simulink model "Empty_Model"  (R2024b)
settings: Solver=FixedStepDiscrete  StartTime=0.0  StopTime=inf  FixedStep=0.01  RelTol=1e-3
libraries: simulink x3, Lib_Model x3
settings Model: PacingRate=0.250000  Creator=HHI  LastModifiedBy=HHI

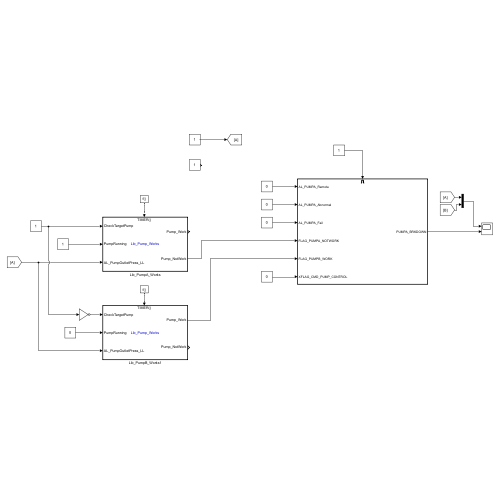
[thumbnail: Simulink's stored preview of the top-level diagram]
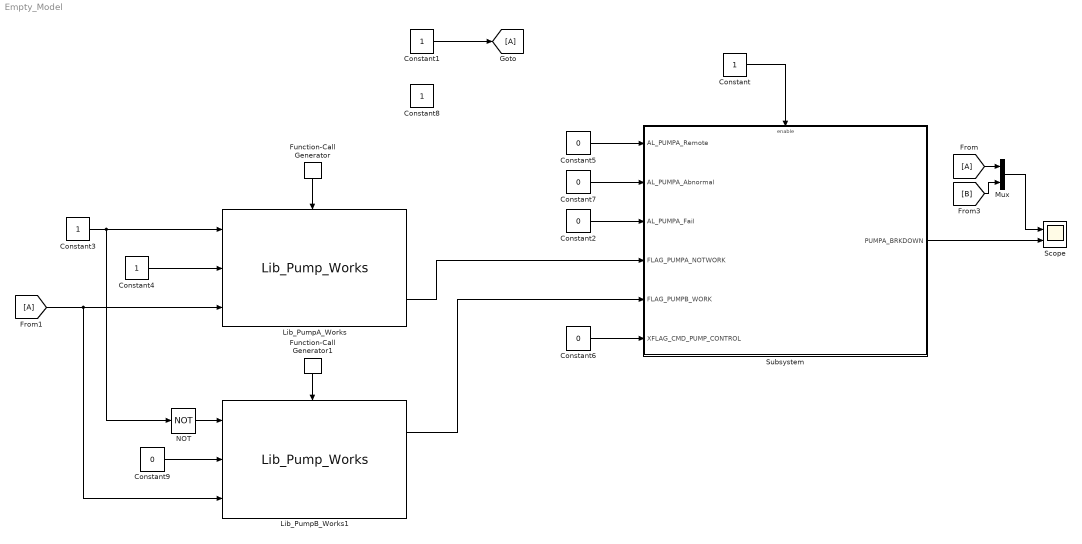
== system Empty_Model ==
  Constant{,1,3..4,8} (5 alike) : Constant  OutDataTypeStr=boolean
  Constant{2,5..7,9} (5 alike) : Constant  Value=0  OutDataTypeStr=boolean
  From : From
  From1 : From
  Function-Call Generator : simulink/Ports & Subsystems/Function-Call Generator  sample_time=1  numberOfIterations=1  DisallowWideOutput=off
  Function-Call Generator1 : simulink/Ports & Subsystems/Function-Call Generator  sample_time=1  numberOfIterations=1  DisallowWideOutput=off
  Goto : Goto
  Lib_PumpA_Works : Lib_Model/Lib_Pump_Works  SystemSampleTime=-1  VariantActivationTime=update diagram  AllowFlexibleInterface=on  Latency=0  AutoFrameSizeCalculation=off
  Lib_PumpB_Works1 : Lib_Model/Lib_Pump_Works  SystemSampleTime=-1  VariantActivationTime=update diagram  AllowFlexibleInterface=on  Latency=0  AutoFrameSizeCalculation=off
  Mux : Mux  Inputs=2
  NOT : Logic  Operator=NOT  IconShape=distinctive  AllPortsSameDT=off  OutDataTypeStr=boolean
  Scope : Scope  NumInputPorts=2
  Subsystem : Subsystem
  wires:
  Constant2/1 -> Subsystem/3(AL_PUMPA_Fail)
  Constant6/1 -> Subsystem/6(XFLAG_CMD_PUMP_CONTROL)
  Subsystem/1(PUMPA_BRKDOWN) -> Scope/2
  Constant1/1 -> Goto/1
  From/1 -> Mux/1
  Constant/1 -> Subsystem/Enable
  Constant7/1 -> Subsystem/2(AL_PUMPA_Abnormal)
  Constant5/1 -> Subsystem/1(AL_PUMPA_Remote)
  Function-Call Generator/1 -> Lib_PumpA_Works/Trigger
  Function-Call Generator1/1 -> Lib_PumpB_Works1/Trigger
  From1/1 -> Lib_PumpB_Works1/3, Lib_PumpA_Works/3
  Constant4/1 -> Lib_PumpA_Works/2
  NOT/1 -> Lib_PumpB_Works1/1
  Constant3/1 -> NOT/1, Lib_PumpA_Works/1
  Lib_PumpA_Works/2 -> Subsystem/4(FLAG_PUMPA_NOTWORK)
  Lib_PumpB_Works1/1 -> Subsystem/5(FLAG_PUMPB_WORK)
  Mux/1 -> Scope/1
  [B] -> Mux/2
  Constant9/1 -> Lib_PumpB_Works1/2

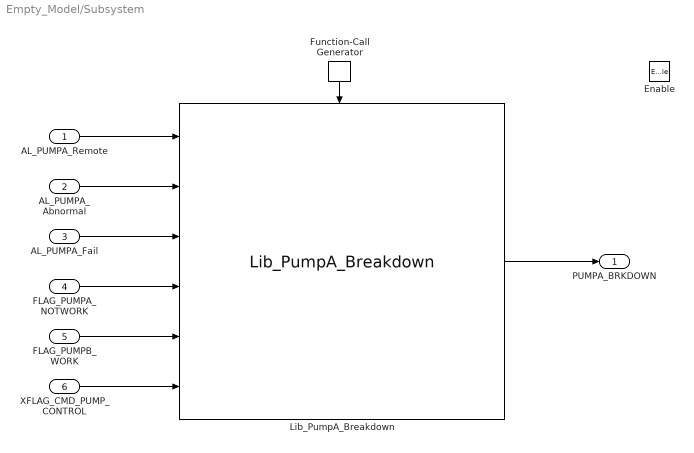
== system Empty_Model/Subsystem ==
  AL_PUMPA_Remote : Inport
  AL_PUMPA_Abnormal : Inport  Port=2
  AL_PUMPA_Fail : Inport  Port=3
  FLAG_PUMPA_NOTWORK : Inport  Port=4
  FLAG_PUMPB_WORK : Inport  Port=5
  XFLAG_CMD_PUMP_CONTROL : Inport  Port=6
  Enable : EnablePort
  Function-Call Generator : simulink/Ports & Subsystems/Function-Call Generator  sample_time=1  numberOfIterations=1  DisallowWideOutput=off
  Lib_PumpA_Breakdown : Lib_Model/Lib_PumpA_Breakdown  SystemSampleTime=-1  VariantActivationTime=update diagram  AllowFlexibleInterface=on  Latency=0  AutoFrameSizeCalculation=off
  PUMPA_BRKDOWN : Outport
  wires:
  AL_PUMPA_Fail/1 -> Lib_PumpA_Breakdown/3
  AL_PUMPA_Remote/1 -> Lib_PumpA_Breakdown/1
  Lib_PumpA_Breakdown/1 -> PUMPA_BRKDOWN/1
  Function-Call Generator/1 -> Lib_PumpA_Breakdown/Trigger
  XFLAG_CMD_PUMP_CONTROL/1 -> Lib_PumpA_Breakdown/6
  AL_PUMPA_Abnormal/1 -> Lib_PumpA_Breakdown/2
  FLAG_PUMPA_NOTWORK/1 -> Lib_PumpA_Breakdown/4
  FLAG_PUMPB_WORK/1 -> Lib_PumpA_Breakdown/5
